simulink model "exampleSMC"  (R2018b)
settings: Solver=VariableStepAuto  StartTime=0.0  StopTime=10.0  RelTol=1e-3
settings Model: Creator=zhiqi  LastModifiedBy=zhiqi

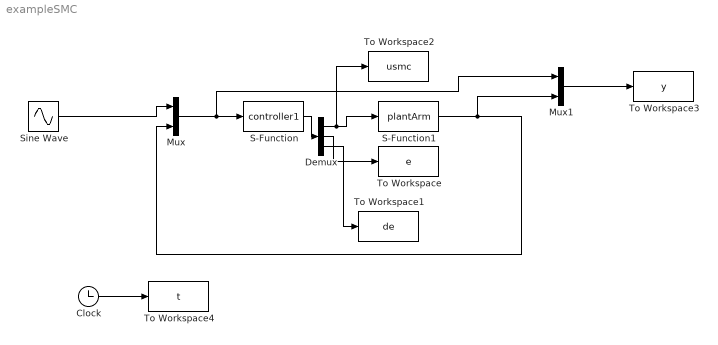
== system exampleSMC ==
  Clock : Clock
  Demux : Demux  Outputs=3
  Mux : Mux  Inputs=2
  Mux1 : Mux  Inputs=2
  S-Function : S-Function  FunctionName=controller1  SFunctionDeploymentMode=off  EnableBusSupport=off
  S-Function1 : S-Function  FunctionName=plantArm  SFunctionDeploymentMode=off  EnableBusSupport=off
  Sine Wave : Sin  Amplitude=0.03  Bias=0.06  Frequency=0.1  SampleTime=0
  To Workspace : ToWorkspace  VariableName=e  SaveFormat=Timeseries  SampleTime=-1
  To Workspace1 : ToWorkspace  VariableName=de  SaveFormat=Timeseries  SampleTime=-1
  To Workspace2 : ToWorkspace  VariableName=usmc  SaveFormat=Timeseries  SampleTime=-1
  To Workspace3 : ToWorkspace  VariableName=y  SaveFormat=Timeseries  SampleTime=-1
  To Workspace4 : ToWorkspace  VariableName=t  SaveFormat=Timeseries  SampleTime=-1
  wires:
  Sine Wave/1 -> Mux/1
  Mux/1 -> Mux1/1, S-Function/1
  S-Function1/1 -> Mux1/2, Mux/2
  S-Function/1 -> Demux/1
  Demux/1 -> To Workspace2/1, S-Function1/1
  Demux/2 -> To Workspace/1
  Demux/3 -> To Workspace1/1
  Mux1/1 -> To Workspace3/1
  Clock/1 -> To Workspace4/1
